simulink model "cps_4_13a"  (R2016a)
settings: Solver=FixedStepAuto  StartTime=0.0  StopTime=10.0  FixedStep=0.01  RelTol=1e-3
libraries: simulink x21
settings Model: Creator=benyett  LastModifiedBy=yettbh

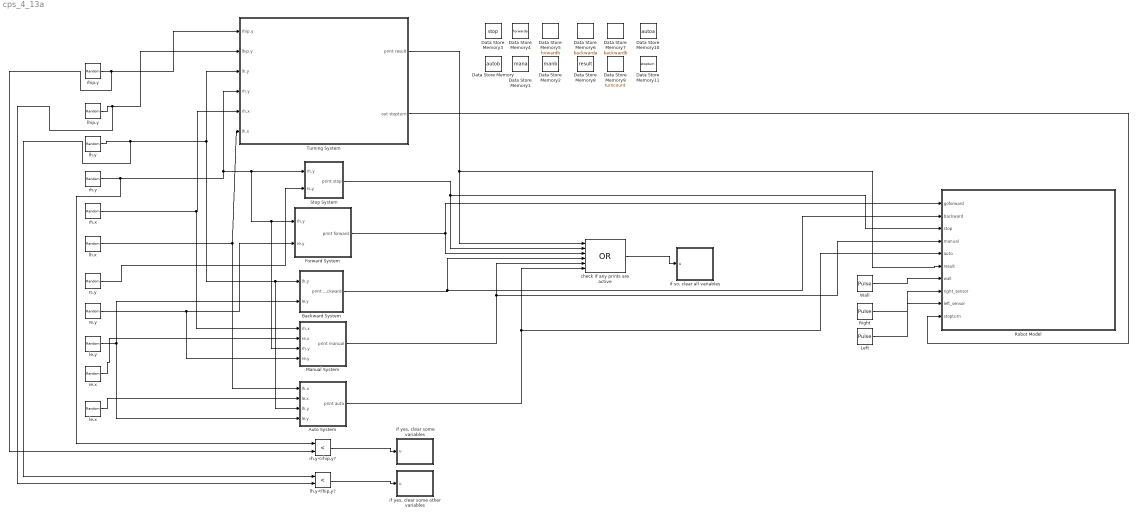
== system cps_4_13a ==
  Auto System : Subsystem
  Backward System : Subsystem
  Data Store Memory : DataStoreMemory  DataStoreName=autob  ReadBeforeWriteMsg=warning  WriteAfterWriteMsg=warning  WriteAfterReadMsg=warning  ShowAdditionalParam=off  OutDataTypeStr=double
  Data Store Memory1 : DataStoreMemory  DataStoreName=mana  ReadBeforeWriteMsg=warning  WriteAfterWriteMsg=warning  WriteAfterReadMsg=warning  ShowAdditionalParam=off  OutDataTypeStr=double
  Data Store Memory10 : DataStoreMemory  DataStoreName=autoa  ReadBeforeWriteMsg=warning  WriteAfterWriteMsg=warning  WriteAfterReadMsg=warning  ShowAdditionalParam=off  OutDataTypeStr=double
  Data Store Memory11 : DataStoreMemory  DataStoreName=stopturn  ReadBeforeWriteMsg=warning  WriteAfterWriteMsg=warning  WriteAfterReadMsg=warning  ShowAdditionalParam=off  OutDataTypeStr=double
  Data Store Memory2 : DataStoreMemory  DataStoreName=manb  ReadBeforeWriteMsg=warning  WriteAfterWriteMsg=warning  WriteAfterReadMsg=warning  ShowAdditionalParam=off  OutDataTypeStr=double
  Data Store Memory3 : DataStoreMemory  DataStoreName=stop  ReadBeforeWriteMsg=warning  WriteAfterWriteMsg=warning  WriteAfterReadMsg=warning  ShowAdditionalParam=off  OutDataTypeStr=double
  Data Store Memory4 : DataStoreMemory  DataStoreName=forwarda  ReadBeforeWriteMsg=warning  WriteAfterWriteMsg=warning  WriteAfterReadMsg=warning  ShowAdditionalParam=off  OutDataTypeStr=double
  Data Store Memory5 : DataStoreMemory  DataStoreName=forwardb  ReadBeforeWriteMsg=warning  WriteAfterWriteMsg=warning  WriteAfterReadMsg=warning  ShowAdditionalParam=off  OutDataTypeStr=double
  Data Store Memory6 : DataStoreMemory  DataStoreName=backwarda  ReadBeforeWriteMsg=warning  WriteAfterWriteMsg=warning  WriteAfterReadMsg=warning  ShowAdditionalParam=off  OutDataTypeStr=double
  Data Store Memory7 : DataStoreMemory  DataStoreName=backwardb  ReadBeforeWriteMsg=warning  WriteAfterWriteMsg=warning  WriteAfterReadMsg=warning  ShowAdditionalParam=off  OutDataTypeStr=double
  Data Store Memory8 : DataStoreMemory  DataStoreName=result  ReadBeforeWriteMsg=warning  WriteAfterWriteMsg=warning  WriteAfterReadMsg=warning  ShowAdditionalParam=off  OutDataTypeStr=double
  Data Store Memory9 : DataStoreMemory  DataStoreName=turncount  ReadBeforeWriteMsg=warning  WriteAfterWriteMsg=warning  WriteAfterReadMsg=warning  ShowAdditionalParam=off  OutDataTypeStr=double
  Forward System : Subsystem
  Left : DiscretePulseGenerator  PulseType=Time based  Period=10  PulseWidth=10  PhaseDelay=7.5
  Manual System : Subsystem
  Right : DiscretePulseGenerator  PulseType=Time based  Period=10  PulseWidth=10  PhaseDelay=4
  Robot Model : Stateflow chart  TreatAsAtomicUnit=on
  Stop System : Subsystem
  Turning System : Subsystem
  Wall : DiscretePulseGenerator  PulseType=Time based  Period=10  PulseWidth=10
  check if any prints are active : Logic  Operator=OR  Inputs=6  AllPortsSameDT=off  OutDataTypeStr=boolean
  "if so, clear all variables" : MATLAB Function  TreatAsAtomicUnit=on
  "if yes, clear some other variables" : MATLAB Function  TreatAsAtomicUnit=on
  "if yes, clear some variables" : MATLAB Function  TreatAsAtomicUnit=on
  le.x : RandomNumber  Seed=10  SampleTime=0.01
  le.y : RandomNumber  Seed=8  SampleTime=0.01
  lh.x : RandomNumber  Seed=5  SampleTime=0.01
  lh.y : RandomNumber  Seed=2  SampleTime=0.01
  lh.y<lhip.y? : RelationalOperator  Operator=<  OutDataTypeStr=boolean
  lhip.y : RandomNumber  Seed=1  SampleTime=0.01
  re.x : RandomNumber  Seed=9  SampleTime=0.01
  re.y : RandomNumber  Seed=7  SampleTime=0.01
  rh.x : RandomNumber  Seed=4  SampleTime=0.01
  rh.y : RandomNumber  Seed=3  SampleTime=0.01
  rh.y<rhip.y? : RelationalOperator  Operator=<  OutDataTypeStr=boolean
  rhip.y : RandomNumber  SampleTime=0.01
  rs.y : RandomNumber  Seed=6  SampleTime=0.01
  wires:
  Turning System/1(print result) -> Robot Model/6(result), check if any prints are active/1
  Stop System/1(print stop) -> Robot Model/3(stop), check if any prints are active/2
  Forward System/1(print forward) -> Robot Model/1(goforward), check if any prints are active/3
  Backward System/1(print backward) -> Robot Model/2(backward), check if any prints are active/4
  Manual System/1(print manual) -> Robot Model/4(manual), check if any prints are active/5
  Auto System/1(print auto) -> Robot Model/5(auto), check if any prints are active/6
  check if any prints are active/1 -> "if so, clear all variables"/1(u)
  rhip.y/1 -> rh.y<rhip.y?/2, Turning System/1(rhip.y)
  lhip.y/1 -> lh.y<lhip.y?/2, Turning System/2(lhip.y)
  lh.y/1 -> lh.y<lhip.y?/1, Auto System/3(lh.y), Backward System/1(lh.y), Turning System/3(lh.y)
  rh.y/1 -> Manual System/3(rh.y), Forward System/1(rh.y), Stop System/1(rh.y), Turning System/4(rh.y), rh.y<rhip.y?/1
  rh.x/1 -> Manual System/1(rh.x), Turning System/5(rh.x)
  lh.x/1 -> Auto System/1(lh.x), Turning System/6(lh.x)
  rs.y/1 -> Stop System/2(rs.y)
  re.y/1 -> Manual System/4(re.y), Forward System/2(re.y)
  le.y/1 -> Auto System/4(le.y), Backward System/2(le.y)
  re.x/1 -> Manual System/2(re.x)
  le.x/1 -> Auto System/2(le.x)
  Wall/1 -> Robot Model/7(wall)
  Right/1 -> Robot Model/8(right_sensor)
  Left/1 -> Robot Model/9(left_sensor)
  rh.y<rhip.y?/1 -> "if yes, clear some variables"/1(u)
  lh.y<lhip.y?/1 -> "if yes, clear some other variables"/1(u)
  Turning System/2(out stopturn) -> Robot Model/10(stopturn)

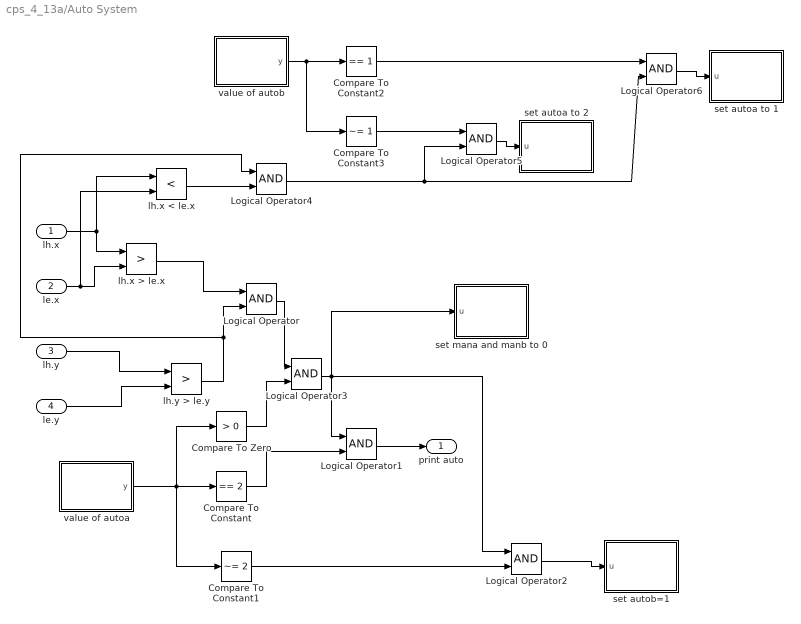
== system cps_4_13a/Auto System ==
  lh.x : Inport
  le.x : Inport  Port=2
  lh.y : Inport  Port=3
  le.y : Inport  Port=4
  Compare To Constant : simulink/Logic and Bit Operations/Compare To Constant  relop===  const=2  OutDataTypeStr=boolean
  Compare To Constant1 : simulink/Logic and Bit Operations/Compare To Constant  relop=~=  const=2  OutDataTypeStr=boolean
  Compare To Constant2 : simulink/Logic and Bit Operations/Compare To Constant  relop===  const=1  OutDataTypeStr=boolean
  Compare To Constant3 : simulink/Logic and Bit Operations/Compare To Constant  relop=~=  const=1  OutDataTypeStr=boolean
  Compare To Zero : simulink/Logic and Bit Operations/Compare To Zero  relop=>  OutDataTypeStr=boolean
  Logical Operator{,1..6} (7 alike) : Logic  AllPortsSameDT=off  OutDataTypeStr=boolean
  lh.x < le.x : RelationalOperator  Operator=<  OutDataTypeStr=boolean
  lh.x > le.x : RelationalOperator  Operator=>  OutDataTypeStr=boolean
  lh.y > le.y : RelationalOperator  Operator=>  OutDataTypeStr=boolean
  set autoa to 1 : MATLAB Function  TreatAsAtomicUnit=on
  set autoa to 2 : MATLAB Function  TreatAsAtomicUnit=on
  set autob=1 : MATLAB Function  TreatAsAtomicUnit=on
  set mana and manb to 0 : MATLAB Function  TreatAsAtomicUnit=on
  value of autoa : MATLAB Function  TreatAsAtomicUnit=on
  value of autob : MATLAB Function  TreatAsAtomicUnit=on
  print auto : Outport
  wires:
  le.x/1 -> lh.x < le.x/2, lh.x > le.x/2
  lh.x/1 -> lh.x < le.x/1, lh.x > le.x/1
  le.y/1 -> lh.y > le.y/2
  lh.y/1 -> lh.y > le.y/1
  lh.x > le.x/1 -> Logical Operator/1
  lh.y > le.y/1 -> Logical Operator4/1, Logical Operator/2
  Logical Operator/1 -> Logical Operator3/1
  value of autoa/1(y) -> Compare To Zero/1, Compare To Constant1/1, Compare To Constant/1
  Compare To Constant/1 -> Logical Operator1/2
  Compare To Constant1/1 -> Logical Operator2/2
  Logical Operator1/1 -> print auto/1
  Logical Operator2/1 -> set autob=1/1(u)
  Logical Operator3/1 -> set mana and manb to 0/1(u), Logical Operator1/1, Logical Operator2/1
  Compare To Zero/1 -> Logical Operator3/2
  lh.x < le.x/1 -> Logical Operator4/2
  value of autob/1(y) -> Compare To Constant3/1, Compare To Constant2/1
  Compare To Constant3/1 -> Logical Operator5/1
  Compare To Constant2/1 -> Logical Operator6/1
  Logical Operator4/1 -> Logical Operator5/2, Logical Operator6/2
  Logical Operator5/1 -> set autoa to 2/1(u)
  Logical Operator6/1 -> set autoa to 1/1(u)

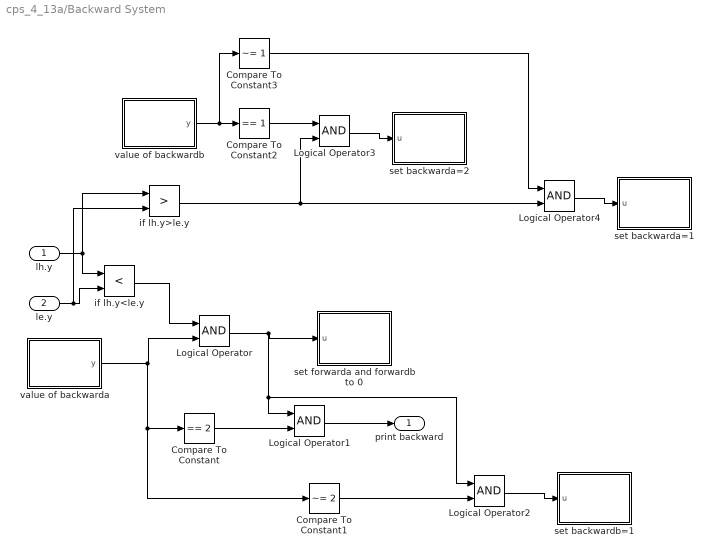
== system cps_4_13a/Backward System ==
  lh.y : Inport
  le.y : Inport  Port=2
  Compare To Constant : simulink/Logic and Bit Operations/Compare To Constant  relop===  const=2  OutDataTypeStr=boolean
  Compare To Constant1 : simulink/Logic and Bit Operations/Compare To Constant  relop=~=  const=2  OutDataTypeStr=boolean
  Compare To Constant2 : simulink/Logic and Bit Operations/Compare To Constant  relop===  const=1  OutDataTypeStr=boolean
  Compare To Constant3 : simulink/Logic and Bit Operations/Compare To Constant  relop=~=  const=1  OutDataTypeStr=boolean
  Logical Operator{,1..4} (5 alike) : Logic  AllPortsSameDT=off  OutDataTypeStr=boolean
  if lh.y<le.y : RelationalOperator  Operator=<  OutDataTypeStr=boolean
  if lh.y>le.y : RelationalOperator  Operator=>  OutDataTypeStr=boolean
  set backwarda=1 : MATLAB Function  TreatAsAtomicUnit=on
  set backwarda=2 : MATLAB Function  TreatAsAtomicUnit=on
  set backwardb=1 : MATLAB Function  TreatAsAtomicUnit=on
  set forwarda and forwardb to 0 : MATLAB Function  TreatAsAtomicUnit=on
  value of backwarda : MATLAB Function  TreatAsAtomicUnit=on
  value of backwardb : MATLAB Function  TreatAsAtomicUnit=on
  print backward : Outport
  wires:
  le.y/1 -> if lh.y>le.y/2, if lh.y<le.y/2
  lh.y/1 -> if lh.y>le.y/1, if lh.y<le.y/1
  if lh.y<le.y/1 -> Logical Operator/1
  value of backwarda/1(y) -> Compare To Constant1/1, Compare To Constant/1, Logical Operator/2
  Logical Operator/1 -> Logical Operator2/1, Logical Operator1/1, set forwarda and forwardb to 0/1(u)
  Compare To Constant/1 -> Logical Operator1/2
  Logical Operator1/1 -> print backward/1
  Compare To Constant1/1 -> Logical Operator2/2
  Logical Operator2/1 -> set backwardb=1/1(u)
  value of backwardb/1(y) -> Compare To Constant3/1, Compare To Constant2/1
  if lh.y>le.y/1 -> Logical Operator3/2, Logical Operator4/2
  Compare To Constant2/1 -> Logical Operator3/1
  Compare To Constant3/1 -> Logical Operator4/1
  Logical Operator4/1 -> set backwarda=1/1(u)
  Logical Operator3/1 -> set backwarda=2/1(u)

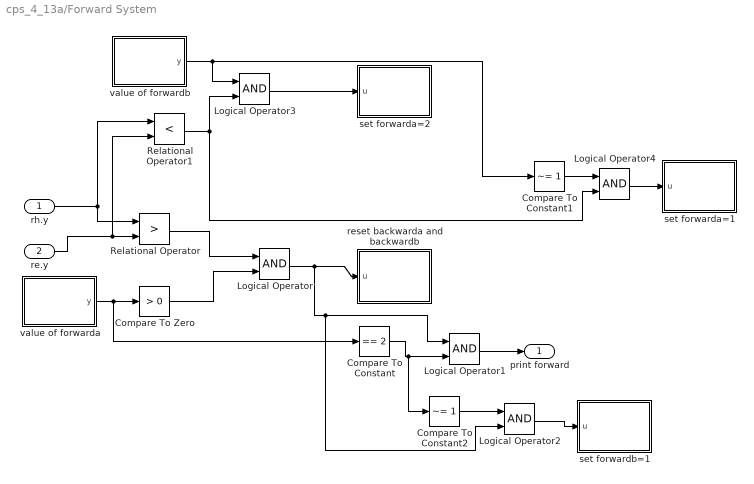
== system cps_4_13a/Forward System ==
  rh.y : Inport
  re.y : Inport  Port=2
  Compare To Constant : simulink/Logic and Bit Operations/Compare To Constant  relop===  const=2  OutDataTypeStr=boolean
  Compare To Constant1 : simulink/Logic and Bit Operations/Compare To Constant  relop=~=  const=1  OutDataTypeStr=boolean
  Compare To Constant2 : simulink/Logic and Bit Operations/Compare To Constant  relop=~=  const=1  OutDataTypeStr=boolean
  Compare To Zero : simulink/Logic and Bit Operations/Compare To Zero  relop=>  OutDataTypeStr=boolean
  Logical Operator{,1..4} (5 alike) : Logic  AllPortsSameDT=off  OutDataTypeStr=boolean
  Relational Operator : RelationalOperator  Operator=>  OutDataTypeStr=boolean
  Relational Operator1 : RelationalOperator  Operator=<  OutDataTypeStr=boolean
  reset backwarda and backwardb : MATLAB Function  TreatAsAtomicUnit=on
  set forwarda=1 : MATLAB Function  TreatAsAtomicUnit=on
  set forwarda=2 : MATLAB Function  TreatAsAtomicUnit=on
  set forwardb=1 : MATLAB Function  TreatAsAtomicUnit=on
  value of forwarda : MATLAB Function  TreatAsAtomicUnit=on
  value of forwardb : MATLAB Function  TreatAsAtomicUnit=on
  print forward : Outport
  wires:
  Compare To Zero/1 -> Logical Operator/2
  value of forwarda/1(y) -> Compare To Constant/1, Compare To Zero/1
  re.y/1 -> Relational Operator1/2, Relational Operator/2
  rh.y/1 -> Relational Operator1/1, Relational Operator/1
  Relational Operator/1 -> Logical Operator/1
  Logical Operator/1 -> Logical Operator2/2, Logical Operator1/1, reset backwarda and backwardb/1(u)
  Compare To Constant/1 -> Compare To Constant2/1, Logical Operator1/2
  Logical Operator1/1 -> print forward/1
  Compare To Constant2/1 -> Logical Operator2/1
  Logical Operator2/1 -> set forwardb=1/1(u)
  value of forwardb/1(y) -> Compare To Constant1/1, Logical Operator3/1
  Relational Operator1/1 -> Logical Operator4/2, Logical Operator3/2
  Logical Operator3/1 -> set forwarda=2/1(u)
  Compare To Constant1/1 -> Logical Operator4/1
  Logical Operator4/1 -> set forwarda=1/1(u)

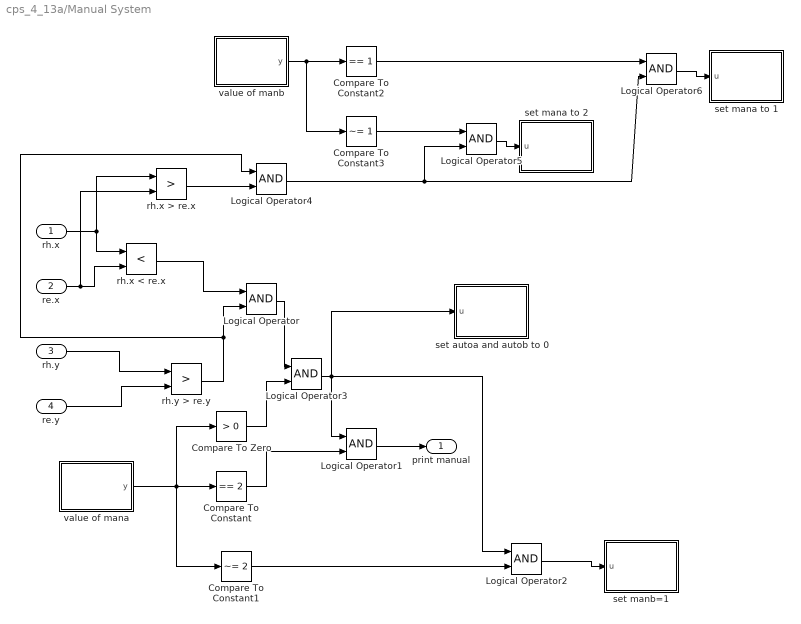
== system cps_4_13a/Manual System ==
  rh.x : Inport
  re.x : Inport  Port=2
  rh.y : Inport  Port=3
  re.y : Inport  Port=4
  Compare To Constant : simulink/Logic and Bit Operations/Compare To Constant  relop===  const=2  OutDataTypeStr=boolean
  Compare To Constant1 : simulink/Logic and Bit Operations/Compare To Constant  relop=~=  const=2  OutDataTypeStr=boolean
  Compare To Constant2 : simulink/Logic and Bit Operations/Compare To Constant  relop===  const=1  OutDataTypeStr=boolean
  Compare To Constant3 : simulink/Logic and Bit Operations/Compare To Constant  relop=~=  const=1  OutDataTypeStr=boolean
  Compare To Zero : simulink/Logic and Bit Operations/Compare To Zero  relop=>  OutDataTypeStr=boolean
  Logical Operator{,1..6} (7 alike) : Logic  AllPortsSameDT=off  OutDataTypeStr=boolean
  rh.x < re.x : RelationalOperator  Operator=<  OutDataTypeStr=boolean
  rh.x > re.x : RelationalOperator  Operator=>  OutDataTypeStr=boolean
  rh.y > re.y : RelationalOperator  Operator=>  OutDataTypeStr=boolean
  set autoa and autob to 0 : MATLAB Function  TreatAsAtomicUnit=on
  set mana to 1 : MATLAB Function  TreatAsAtomicUnit=on
  set mana to 2 : MATLAB Function  TreatAsAtomicUnit=on
  set manb=1 : MATLAB Function  TreatAsAtomicUnit=on
  value of mana : MATLAB Function  TreatAsAtomicUnit=on
  value of manb : MATLAB Function  TreatAsAtomicUnit=on
  print manual : Outport
  wires:
  Logical Operator6/1 -> set mana to 1/1(u)
  Logical Operator5/1 -> set mana to 2/1(u)
  Logical Operator4/1 -> Logical Operator6/2, Logical Operator5/2
  Compare To Constant2/1 -> Logical Operator6/1
  Compare To Constant3/1 -> Logical Operator5/1
  value of manb/1(y) -> Compare To Constant2/1, Compare To Constant3/1
  rh.x > re.x/1 -> Logical Operator4/2
  Compare To Zero/1 -> Logical Operator3/2
  Logical Operator3/1 -> Logical Operator2/1, Logical Operator1/1, set autoa and autob to 0/1(u)
  Logical Operator2/1 -> set manb=1/1(u)
  Logical Operator1/1 -> print manual/1
  Compare To Constant1/1 -> Logical Operator2/2
  Compare To Constant/1 -> Logical Operator1/2
  value of mana/1(y) -> Compare To Constant/1, Compare To Constant1/1, Compare To Zero/1
  Logical Operator/1 -> Logical Operator3/1
  rh.y > re.y/1 -> Logical Operator/2, Logical Operator4/1
  rh.x < re.x/1 -> Logical Operator/1
  rh.y/1 -> rh.y > re.y/1
  re.y/1 -> rh.y > re.y/2
  rh.x/1 -> rh.x < re.x/1, rh.x > re.x/1
  re.x/1 -> rh.x < re.x/2, rh.x > re.x/2

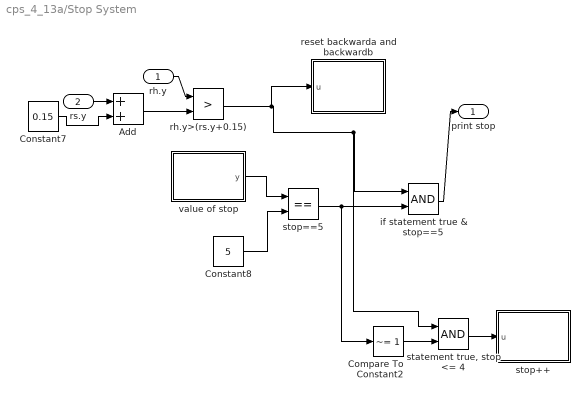
== system cps_4_13a/Stop System ==
  rh.y : Inport
  rs.y : Inport  Port=2
  Add : Sum
  Compare To Constant2 : simulink/Logic and Bit Operations/Compare To Constant  relop=~=  const=1  OutDataTypeStr=boolean
  Constant7 : Constant  Value=0.15
  Constant8 : Constant  Value=5
  if statement true & stop==5 : Logic  AllPortsSameDT=off  OutDataTypeStr=boolean
  reset backwarda and backwardb : MATLAB Function  TreatAsAtomicUnit=on
  rh.y>(rs.y+0.15) : RelationalOperator  Operator=>  OutDataTypeStr=boolean
  "statement true, stop <= 4" : Logic  AllPortsSameDT=off  OutDataTypeStr=boolean
  stop++ : MATLAB Function  TreatAsAtomicUnit=on
  stop==5 : RelationalOperator  Operator===  OutDataTypeStr=boolean
  value of stop : MATLAB Function  TreatAsAtomicUnit=on
  print stop : Outport
  wires:
  stop==5/1 -> Compare To Constant2/1, if statement true & stop==5/2
  rs.y/1 -> Add/1
  Add/1 -> rh.y>(rs.y+0.15)/2
  Constant7/1 -> Add/2
  rh.y/1 -> rh.y>(rs.y+0.15)/1
  value of stop/1(y) -> stop==5/1
  Constant8/1 -> stop==5/2
  rh.y>(rs.y+0.15)/1 -> reset backwarda and backwardb/1(u), "statement true, stop <= 4"/1, if statement true & stop==5/1
  if statement true & stop==5/1 -> print stop/1
  Compare To Constant2/1 -> "statement true, stop <= 4"/2
  "statement true, stop <= 4"/1 -> stop++/1(u)

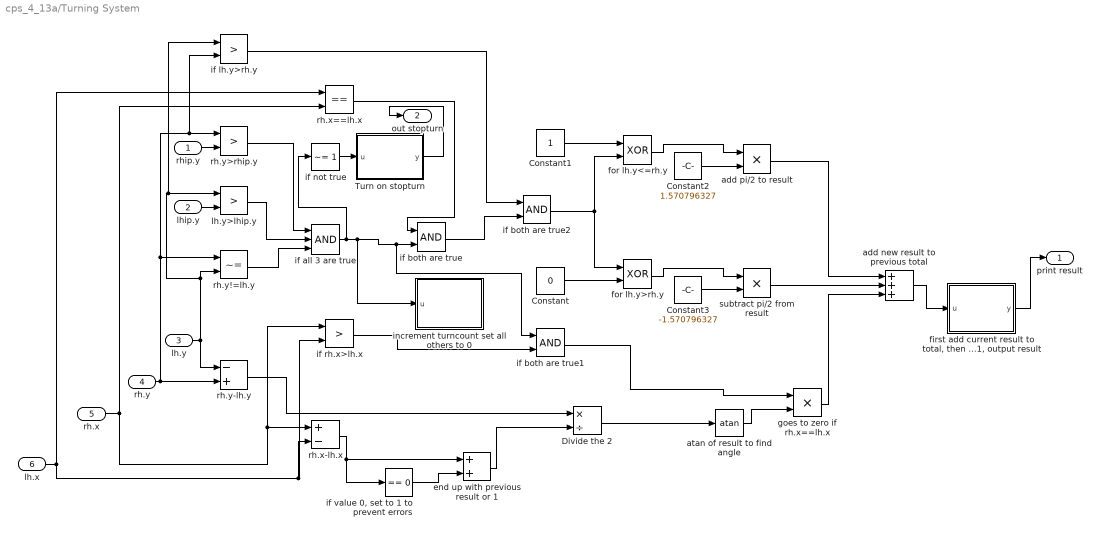
== system cps_4_13a/Turning System ==
  rhip.y : Inport
  lhip.y : Inport  Port=2
  lh.y : Inport  Port=3
  rh.y : Inport  Port=4
  rh.x : Inport  Port=5
  lh.x : Inport  Port=6
  Constant : Constant  Value=0
  Constant1 : Constant
  Constant2 : Constant  Value=1.570796327
  Constant3 : Constant  Value=-1.570796327
  Divide the 2 : Product  Inputs=*/
  Turn on stopturn : MATLAB Function  TreatAsAtomicUnit=on
  add new result to previous total : Sum  Inputs=+++
  add pi/2 to result : Product
  atan of result to find angle : Trigonometry  Operator=atan
  end up with previous result or 1 : Sum
  "first add current result to total, then if turncount==1, output result " : MATLAB Function  TreatAsAtomicUnit=on
  for lh.y<=rh.y : Logic  Operator=XOR  AllPortsSameDT=off  OutDataTypeStr=boolean
  for lh.y>rh.y : Logic  Operator=XOR  AllPortsSameDT=off  OutDataTypeStr=boolean
  goes to zero if rh.x==lh.x : Product
  if all 3 are true : Logic  Inputs=3  AllPortsSameDT=off  OutDataTypeStr=boolean
  if both are true : Logic  AllPortsSameDT=off  OutDataTypeStr=boolean
  if both are true1 : Logic  AllPortsSameDT=off  OutDataTypeStr=boolean
  if both are true2 : Logic  AllPortsSameDT=off  OutDataTypeStr=boolean
  if lh.y>rh.y : RelationalOperator  Operator=>  OutDataTypeStr=boolean
  if not true : simulink/Logic and Bit Operations/Compare To Constant  relop=~=  const=1  OutDataTypeStr=boolean
  if rh.x>lh.x : RelationalOperator  Operator=>  OutDataTypeStr=boolean
  "if value 0, set to 1 to prevent errors" : simulink/Logic and Bit Operations/Compare To Zero  relop===  OutDataTypeStr=boolean
  increment turncount set all others to 0 : MATLAB Function  TreatAsAtomicUnit=on
  lh.y>lhip.y : RelationalOperator  Operator=>  OutDataTypeStr=boolean
  rh.x-lh.x : Sum  Inputs=+-
  rh.x==lh.x : RelationalOperator  Operator===  OutDataTypeStr=boolean
  rh.y!=lh.y : RelationalOperator  Operator=~=  OutDataTypeStr=boolean
  rh.y-lh.y : Sum  Inputs=-+
  rh.y>rhip.y : RelationalOperator  Operator=>  OutDataTypeStr=boolean
  subtract pi/2 from result : Product
  print result : Outport
  out stopturn : Outport  Port=2
  wires:
  rhip.y/1 -> rh.y>rhip.y/2
  rh.x/1 -> rh.x==lh.x/2, if rh.x>lh.x/1, rh.x-lh.x/1
  lh.x/1 -> rh.x==lh.x/1, if rh.x>lh.x/2, rh.x-lh.x/2
  "first add current result to total, then if turncount==1, output result "/1(y) -> print result/1
  lhip.y/1 -> lh.y>lhip.y/2
  lh.y/1 -> rh.y!=lh.y/2, if lh.y>rh.y/1, lh.y>lhip.y/1, rh.y-lh.y/1
  rh.y/1 -> if lh.y>rh.y/2, rh.y>rhip.y/1, rh.y!=lh.y/1, rh.y-lh.y/2
  rh.y>rhip.y/1 -> if all 3 are true/1
  lh.y>lhip.y/1 -> if all 3 are true/2
  rh.y!=lh.y/1 -> if all 3 are true/3
  rh.x==lh.x/1 -> if both are true/1
  if all 3 are true/1 -> if not true/1, increment turncount set all others to 0/1(u), if both are true1/1, if both are true/2
  if both are true/1 -> if both are true2/2
  if lh.y>rh.y/1 -> if both are true2/1
  Constant1/1 -> for lh.y<=rh.y/1
  if both are true2/1 -> for lh.y>rh.y/1, for lh.y<=rh.y/2
  Constant/1 -> for lh.y>rh.y/2
  for lh.y>rh.y/1 -> subtract pi/2 from result/1
  Constant3/1 -> subtract pi/2 from result/2
  for lh.y<=rh.y/1 -> add pi/2 to result/1
  Constant2/1 -> add pi/2 to result/2
  if rh.x>lh.x/1 -> if both are true1/2
  rh.y-lh.y/1 -> Divide the 2/1
  Divide the 2/1 -> atan of result to find angle/1
  if both are true1/1 -> goes to zero if rh.x==lh.x/1
  atan of result to find angle/1 -> goes to zero if rh.x==lh.x/2
  add pi/2 to result/1 -> add new result to previous total/1
  subtract pi/2 from result/1 -> add new result to previous total/2
  goes to zero if rh.x==lh.x/1 -> add new result to previous total/3
  add new result to previous total/1 -> "first add current result to total, then if turncount==1, output result "/1(u)
  rh.x-lh.x/1 -> end up with previous result or 1/1, "if value 0, set to 1 to prevent errors"/1
  end up with previous result or 1/1 -> Divide the 2/2
  "if value 0, set to 1 to prevent errors"/1 -> end up with previous result or 1/2
  if not true/1 -> Turn on stopturn/1(u)
  Turn on stopturn/1(y) -> out stopturn/1

== matlab function cps_4_13a/Stop System/value of stop ==
  data: y output; stop data_store_memory
function y = fcn
%#codegen
global stop;
y=stop;

== matlab function cps_4_13a/Stop System/stop++ ==
  data: u input; stop data_store_memory
function fcn(u)
%#codegen
global stop;
stop=stop+u;

== matlab function cps_4_13a/Forward System/value of forwarda ==
  data: y output; forwarda data_store_memory
function y = fcn
%#codegen
global forwarda;
y = forwarda;

== matlab function cps_4_13a/Forward System/reset backwarda and backwardb ==
  data: u input; backwarda data_store_memory; backwardb data_store_memory
function fcn(u)
%#codegen
global backwarda;
global backwardb;
if (u==1)
    backwarda=0;
    backwardb=0;
end

== matlab function cps_4_13a/Forward System/set forwardb=1 ==
  data: u input; forwardb data_store_memory
function fcn(u)
%#codegen
global forwardb;
if u==1
    forwardb=1;
end

== matlab function cps_4_13a/Stop System/reset backwarda and backwardb ==
  data: u input; backwarda data_store_memory; backwardb data_store_memory
function fcn(u)
%#codegen
global backwarda;
global backwardb;
if (u==1)
    backwarda=0;
    backwardb=0;
end

== matlab function cps_4_13a/Forward System/value of forwardb ==
  data: y output; forwardb data_store_memory
function y = fcn
%#codegen
global forwardb;
y = forwardb;

== matlab function cps_4_13a/Forward System/set forwarda=2 ==
  data: u input; forwarda data_store_memory
function fcn(u)
%#codegen
global forwarda;
if u==1
    forwarda=2;
end

== matlab function cps_4_13a/Forward System/set forwarda=1 ==
  data: u input; forwarda data_store_memory
function fcn(u)
%#codegen
global forwarda;
if u==1
    forwarda=1;
end

== matlab function cps_4_13a/Backward System/value of backwarda ==
  data: y output; backwarda data_store_memory
function y = fcn
%#codegen
global backwarda;
y = backwarda;

== matlab function cps_4_13a/Backward System/set forwarda and forwardb to 0 ==
  data: u input; forwarda data_store_memory; forwardb data_store_memory
function fcn(u)
%#codegen
global forwarda;
global forwardb;
if u==1
    forwarda=0;
    forwardb=0;
end

== matlab function cps_4_13a/Backward System/set backwardb=1 ==
  data: u input; backwardb data_store_memory
function fcn(u)
%#codegen
global backwardb;
if u==1
    backwardb=1;
end

== matlab function cps_4_13a/Backward System/value of backwardb ==
  data: y output; backwardb data_store_memory
function y = fcn
%#codegen
global backwardb;
y=backwardb;

== matlab function cps_4_13a/Backward System/set backwarda=2 ==
  data: u input; backwarda data_store_memory
function fcn(u)
%#codegen
global backwarda;
if u==1
    backwarda=2;
end

== matlab function cps_4_13a/Backward System/set backwarda=1 ==
  data: u input; backwarda data_store_memory
function fcn(u)
%#codegen
global backwarda;
if u==1
    backwarda=1;
end

== matlab function cps_4_13a/Auto System/value of autoa ==
  data: y output; autoa data_store_memory
function y = fcn
%#codegen
global autoa;
y=autoa;

== matlab function cps_4_13a/Auto System/set autob=1 ==
  data: u input; autob data_store_memory
function fcn(u)
%#codegen
global autob;
if u==1
    autob=1;
end

== matlab function cps_4_13a/Auto System/set mana and manb to 0 ==
  data: u input; mana data_store_memory; manb data_store_memory
function fcn(u)
%#codegen
global mana;
global manb;
if u==1
    mana=0;
    manb=0;
end

== matlab function cps_4_13a/Auto System/value of autob ==
  data: y output; autob data_store_memory
function y = fcn
%#codegen
global autob;
y = autob;

== matlab function cps_4_13a/Auto System/set autoa to 2 ==
  data: u input; autoa data_store_memory
function fcn(u)
%#codegen
global autoa;
if u==1
    autoa=2;
end

== matlab function cps_4_13a/Auto System/set autoa to 1 ==
  data: u input; autoa data_store_memory
function fcn(u)
%#codegen
global autoa
if u==1
    autoa=1;
end

== matlab function cps_4_13a/Manual System/set mana to 1 ==
  data: u input; mana data_store_memory
function fcn(u)
%#codegen
global mana
if u==1
    mana=1;
end

== matlab function cps_4_13a/Manual System/set mana to 2 ==
  data: u input; mana data_store_memory
function fcn(u)
%#codegen
global mana;
if u==1
    mana=2;
end

== matlab function cps_4_13a/Manual System/set manb=1 ==
  data: u input; manb data_store_memory
function fcn(u)
%#codegen
global manb;
if u==1
    manb=1;
end

== matlab function cps_4_13a/Manual System/set autoa and autob to 0 ==
  data: u input; autoa data_store_memory; autob data_store_memory
function fcn(u)
%#codegen
global autoa;
global autob;
if u==1
    autoa=0;
    autob=0;
end

== matlab function cps_4_13a/Manual System/value of mana ==
  data: y output; mana data_store_memory
function y = fcn
%#codegen
global mana;
y=mana;

== matlab function cps_4_13a/Manual System/value of manb ==
  data: y output; manb data_store_memory
function y = fcn
%#codegen
global manb;
y = manb;

== matlab function cps_4_13a/Turning System/increment turncount set all others to 0 ==
  data: u input; backwarda data_store_memory; backwardb data_store_memory; forwarda data_store_memory; forwardb data_store_memory; autoa data_store_memory; autob data_store_memory; mana data_store_memory; manb data_store_memory; stop data_store_memory; turncount data_store_memory; stopturn data_store_memory
function fcn(u)
%#codegen
global backwarda;
global backwardb;
global forwarda;
global forwardb;
global autoa;
global autob;
global mana;
global manb;
global stop;
global turncount;
global stopturn;
if u==1
    backwarda=0;
    backwardb=0;
    forwarda=0;
    forwardb=0;
    autoa=0;
    autob=0;
    mana=0;
    manb=0;
    stop=0;
    stopturn=0;
    turncount=turncount+1;
end

== matlab function cps_4_13a/Turning System/first add current result to total, then if turncount==1, output result  ==
  data: u input; y output; turncount data_store_memory; result data_store_memory
function y = fcn(u)
%#codegen
global result;
global turncount;
result=result+u;
y=0;
if turncount==1
    y=result;
end

== matlab function cps_4_13a/if so, clear all variables ==
  data: u input; stop data_store_memory; forwarda data_store_memory; forwardb data_store_memory; backwarda data_store_memory; backwardb data_store_memory; autoa data_store_memory; autob data_store_memory; mana data_store_memory; manb data_store_memory; result data_store_memory; turncount data_store_memory; stopturn data_store_memory
function fcn(u)
%#codegen
global stop;
global forwarda;
global forwardb;
global backwarda;
global backwardb;
global autoa;
global autob;
global mana;
global manb;
global result;
global turncount;
global stopturn;
if u==1
    stop = 0;
	forwarda = 0;
	forwardb = 0;
	backwarda = 0;
	backwardb = 0;
	autoa = 0;
	autob = 0;
	mana = 0;
	manb = 0;
	result = 0;
	turncount = 0;
    stopturn=0;
end

== matlab function cps_4_13a/if yes, clear some variables ==
  data: u input; mana data_store_memory; manb data_store_memory; stop data_store_memory; turncount data_store_memory; result data_store_memory
function fcn(u)
%#codegen
global mana;
global manb;
global stop;
global turncount;
global result;
if u==1
    mana=0;
    manb=0;
    stop=0;
    turncount=0;
    result=0;
end

== stateflow chart cps_4_13a/Robot Model ==
  state Manual
    state Avoid_Obstacle
    state Stop
      state Stop
      state TurnL
      state TurnR
      (default) -> Manual.Stop.Stop
      Manual.Stop.Stop -> Manual.Stop.TurnR [order 2] : [result<0]
      Manual.Stop.Stop -> Manual.Stop.TurnL [order 1] : [result>0]
      Manual.Stop.TurnL -> Manual.Stop.Stop [order 1] : [stopturn==1]
      Manual.Stop.TurnR -> Manual.Stop.Stop [order 1] : [stopturn==1]
      Manual.Stop.TurnL -> Manual.Stop.TurnR [order 2] : [result<0]
      Manual.Stop.TurnR -> Manual.Stop.TurnL [order 2] : [result>0]
    state Backward
      state Backward
      state TurnL
      state TurnR
      (default) -> Manual.Backward.Backward
      Manual.Backward.Backward -> Manual.Backward.TurnR [order 2] : [result<0]
      Manual.Backward.Backward -> Manual.Backward.TurnL [order 1] : [result>0]
      Manual.Backward.TurnL -> Manual.Backward.Backward [order 1] : [stopturn==1]
      Manual.Backward.TurnR -> Manual.Backward.Backward [order 1] : [stopturn==1]
      Manual.Backward.TurnL -> Manual.Backward.TurnR [order 2] : [result<0]
      Manual.Backward.TurnR -> Manual.Backward.TurnL [order 2] : [result>0]
    state Forward
      state Forward
      state TurnL
      state TurnR
      (default) -> Manual.Forward.Forward
      Manual.Forward.Forward -> Manual.Forward.TurnR [order 2] : [result<0]
      Manual.Forward.Forward -> Manual.Forward.TurnL [order 1] : [result>0]
      Manual.Forward.TurnL -> Manual.Forward.Forward [order 1] : [stopturn==1]
      Manual.Forward.TurnR -> Manual.Forward.Forward [order 1] : [stopturn==1]
      Manual.Forward.TurnL -> Manual.Forward.TurnR [order 2] : [result<0]
      Manual.Forward.TurnR -> Manual.Forward.TurnL [order 2] : [result>0]
    Manual.Backward -> Avoid_Obstacle [order 1] : [wall==1 || left_sensor==1 || right_sensor==1]
    Manual.Stop -> Avoid_Obstacle [order 1] : [wall==1 || left_sensor==1 || right_sensor==1]
    (default) -> Avoid_Obstacle [order 1] : [wall==1 || left_sensor==1 || right_sensor==1]
    Avoid_Obstacle -> Manual.Stop : [wall==0 && left_sensor==0 && right_sensor==0]
    (default) -> Manual.Stop [order 2]
    Manual.Stop -> Manual.Forward [order 3] : [goforward==1]
    Manual.Backward -> Manual.Stop [order 2] : [stop==1]
    Manual.Forward -> Manual.Stop [order 1] : [stop==1]
    Manual.Stop -> Manual.Backward [order 2] : [backward==1]
    Manual.Backward -> Manual.Forward [order 3] : [goforward==1]
    Manual.Forward -> Manual.Backward [order 2] : [backward==1]
  state Auto
    state Forward
    state Backward
    state TurnL
    state TurnR
    Auto.TurnL -> Auto.Forward [order 1] : [right_sensor==0 && wall==0 && left_sensor==0 && after(50,tick)]
    (default) -> Auto.Forward
    Auto.TurnR -> Auto.Forward [order 1] : [right_sensor==0 && wall==0 && left_sensor==0 && after(50,tick)]
    Auto.Forward -> Auto.Backward : [right_sensor==1 || wall==1 || left_sensor==1]
    Auto.Backward -> Auto.TurnR [order 2] : [after(50,tick)]
    Auto.Backward -> Auto.TurnL [order 1] : [after(50,tick)]
    Auto.TurnR -> Auto.Backward [order 2] : [after(50,tick) && (right_sensor==1 || wall==1 || left_sensor==1)]
    Auto.TurnL -> Auto.Backward [order 2] : [after(50,tick) && (right_sensor==1 || wall==1 || left_sensor==1)]
  (default) -> Manual
  Auto -> Manual : [manual==1 && (wall==0 && left_sensor==0 && right_sensor==0)]
  Manual -> Auto : [auto==1 && (wall==0 && left_sensor==0 && right_sensor==0)]
  data: goforward input; backward input; stop input; manual input; auto input; result input; wall input double size=1; right_sensor input double size=1; left_sensor input double size=1; stopturn input

== matlab function cps_4_13a/if yes, clear some other variables ==
  data: u input; autoa data_store_memory; autob data_store_memory; turncount data_store_memory; result data_store_memory
function fcn(u)
%#codegen
global autoa;
global autob;
global turncount;
global result;
if u==1
    autoa=0;
    autob=0;
    turncount=0;
    result=0;
end

== matlab function cps_4_13a/Turning System/Turn on stopturn ==
  data: u input; stopturn data_store_memory; y output
function y=fcn(u)
%#codegen
y=0;
global stopturn;
if u==1
    stopturn=1;
    y=stopturn;
end
